simulink model "lab4_prepare"  (R2021a)
settings: Solver=VariableStepAuto  StartTime=0.0  StopTime=1.00  RelTol=1e-3
libraries: simulink x1
settings Model: Creator=toe75  LastModifiedBy=toe75

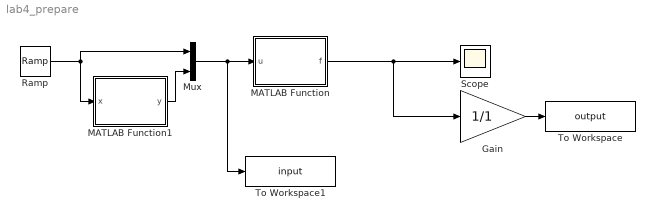
== system lab4_prepare ==
  Gain : Gain  Gain=1/1
  MATLAB Function : MATLAB Function  TreatAsAtomicUnit=on
  MATLAB Function1 : MATLAB Function  TreatAsAtomicUnit=on
  Mux : Mux  Inputs=2
  Ramp : simulink/Sources/Ramp  slope=1  start=0  InitialOutput=0
  Scope : Scope
  To Workspace : ToWorkspace  VariableName=output  SampleTime=-1
  To Workspace1 : ToWorkspace  VariableName=input  SampleTime=-1
  wires:
  Ramp/1 -> MATLAB Function1/1(x), Mux/1
  Mux/1 -> To Workspace1/1, MATLAB Function/1(u)
  MATLAB Function/1(f) -> Scope/1, Gain/1
  Gain/1 -> To Workspace/1
  MATLAB Function1/1(y) -> Mux/2

== matlab function lab4_prepare/MATLAB Function ==
  data: u input; f output
function f = fcn(u)
f = u(1,:)*sin(u(2,:));

== matlab function lab4_prepare/MATLAB Function1 ==
  data: x input; y output
function y = fcn(x)
y = sin(abs(x))+ cos(abs(x));
